simulink model "PX4OutputMappingVtolTailsitter"  (R2026a)
settings: configuration reference "standardSILConfiguraitonParams" (kept outside this file)
undefined symbols (not defined in the file or in its folder): MotorCommandHexBus
settings Model: Creator=Edison Altamirano  LastModifiedBy=Edison Altamirano
settings ConfigSetRef: SourceName=standardSILConfiguraitonParams  SourceLocation=Base Workspace

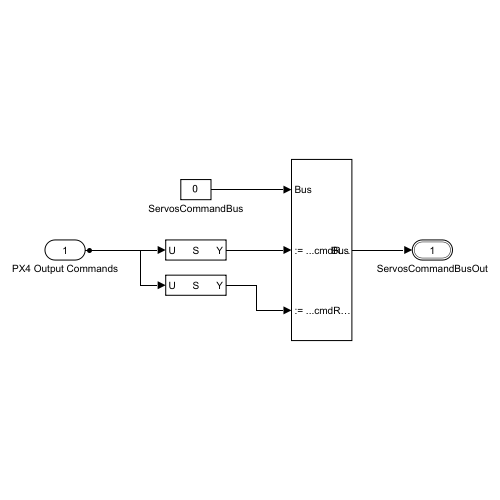
[thumbnail: Simulink's stored preview of the top-level diagram]
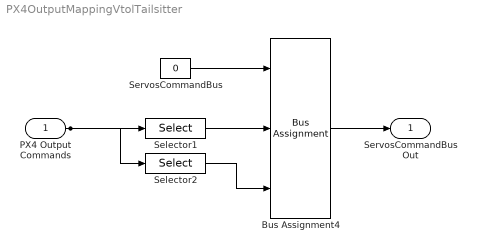
== system PX4OutputMappingVtolTailsitter ==
  PX4 Output Commands : Inport  PortDimensions=16
  Bus Assignment4 : BusAssignment  AssignedSignals=MotorCommandHexBus.cmdRotor1_nd,MotorCommandHexBus.cmdRotor2_nd
  Selector1 : Selector  InputPortWidth=16  IndexOptions=Index vector (dialog)  Indices=1  OutputSizes=1
  Selector2 : Selector  InputPortWidth=16  IndexOptions=Index vector (dialog)  Indices=2  OutputSizes=1
  ServosCommandBus : Constant  Value=0  OutDataTypeStr=Bus: ServosCommandBus
  ServosCommandBusOut : Outport  OutDataTypeStr=Bus: ServosCommandBus
  wires:
  PX4 Output Commands/1 -> Selector1/1, Selector2/1
  Selector1/1 -> Bus Assignment4/2
  ServosCommandBus/1 -> Bus Assignment4/1
  Selector2/1 -> Bus Assignment4/3
  Bus Assignment4/1 -> ServosCommandBusOut/1
